simulink model "stepRecovery_compatibility"  (Simulink 8.3)
settings: Solver=ode3  SolverMode=SingleTasking  StartTime=0.0  StopTime="CONFIG.SIMULATION_TIME "  FixedStep=CONFIG.Ts  RelTol=1e-3
InitFcn:
  | cd(fileparts(which(bdroot)));
  | initStepRecovery;
values from neighbouring files (symbols this model uses):
  baseToWorldRotationPort = '/matlabTorqueBalancing/floatingBaseRotationMatrix:i'    [esperimento_fake2.mat]    (also in initStepRecovery.m = ['/' WBT_modelName '/floatingBaseRotationMatrix:i']; initTorqueBalancing.m = ['/' WBT_modelName '/floatingBaseRotationMatrix:i']; secondo_risultato.mat)
  bVectorConstraints = [0 0 0 0 0 0 0 0 0 0 0 0 ... (19 elements, 19x1)]    [esperimento_fake2.mat]    (also in secondo_risultato.mat)
  CONFIG =     [esperimento_fake2.mat]    (also in secondo_risultato.mat)
  ConstraintsMatrix = [3.73205080757 1 0.267949192431 -0.267949192431 -1 -3.73205080757 -3.73205080757 -1 -0.267949192431 0.267949192431 1 3.73205080757 ... (114 elements, 19x6)]    [esperimento_fake2.mat]    (also in secondo_risultato.mat)
  gain =     [esperimento_fake2.mat]    (also in secondo_risultato.mat)
  references =     [esperimento_fake2.mat]    (also in secondo_risultato.mat)
  reg =     [esperimento_fake2.mat]    (also in secondo_risultato.mat)
  ROBOT_DOF = 23    [esperimento_fake2.mat]    (also in secondo_risultato.mat)
  ROBOT_DOF_FOR_SIMULINK = [1 0 0 0 0 0 0 0 0 0 0 0 ... (529 elements, 23x23)]    [esperimento_fake2.mat]    (also in secondo_risultato.mat)
  sat =     [esperimento_fake2.mat]    (also in secondo_risultato.mat)
  SM =     [esperimento_fake2.mat]    (also in secondo_risultato.mat)
  sm =     [esperimento_fake2.mat]    (also in secondo_risultato.mat)
  WBT_modelName = 'matlabTorqueBalancing'    [esperimento_fake2.mat]    (also in initStepRecovery.m; initTorqueBalancing.m; secondo_risultato.mat)
  WBT_robotName = ''    [esperimento_fake2.mat]    (also in secondo_risultato.mat)
undefined symbols (not defined in the file or in its folder): bVectorConstraintsMPC, ConstraintsMatrixMPC, DiscIntNeverNeededParam, mpc_init
libraries: WBToolboxLibrary x191, simulink x22, simulink_extras x4
(part 5 of 6)

== system stepRecovery_compatibility/DesValues/State Machine Step Recovery/Step Recovery reference generator/Step Recovery Techniques /FPE module ==
  foot_x : Inport
  COM_velocity : Inport  Port=2
  COMx : Inport  Port=3
  Joint Configuration : Inport  Port=4
  Base Pose : Inport  Port=5
  Constraints : Inport  Port=6
  Base Pose1 : InportShadow  Port=5
  "CoM6D ->  CoMXYZ2" : Selector  NumberOfDimensions=2  InputPortWidth=7  IndexOptions=Index vector (dialog),Index vector (dialog)  Indices=[1 2 3],[4]  OutputSizes=1,1
  Constant1 : Constant  Value=9.81
  Constant3 : Constant  Value=CONFIG.SR.FPE.offset
  J_COM : Selector  NumberOfDimensions=2  InputPortWidth=3  IndexOptions=Index vector (dialog),Index vector (dialog)  Indices=[4:6],[4:6]  OutputSizes=1,1
  Joint Configuration1 : InportShadow  Port=4
  MATLAB Function : MATLAB Function  TreatAsAtomicUnit=on
      settings: PermitHierarchicalResolution=ParametersOnly
  MATLAB Function2 : MATLAB Function  TreatAsAtomicUnit=on
      settings: PermitHierarchicalResolution=ParametersOnly
  Mass Matrix : WBToolboxLibrary/wholeBodyModel/Dynamics/Mass Matrix  robotName=WBT_robotName  localName=WBT_modelName  wbiFile=WBT_wbiFilename  wbiList=WBT_wbiList
  Mbb : Selector  NumberOfDimensions=2  InputPortWidth=3  IndexOptions=Index vector (dialog),Index vector (dialog)  Indices=[1:6],[1:6]  OutputSizes=1,1
  Out of left foot_CH : Subsystem
  Scope2 : Scope
      settings: TimeRange=auto  MaxDataPoints=5000  SaveToWorkspace=off  YMin=0.9762  YMax=1.00264  SampleTime=-1
  Switch : Switch  Criteria=u2 > Threshold
  To Workspace : ToWorkspace  VariableName=dissipation  SampleTime=-1
  mass : Selector  NumberOfDimensions=2  InputPortWidth=3  IndexOptions=Index vector (dialog),Index vector (dialog)  Indices=[1],[1]  OutputSizes=1,1
  FPE : Outport
  OUT_L : Outport  Port=2
  Direction : Outport  Port=3
  FPE_ORIGINAL : Outport  Port=4
  theta_bar : Outport  Port=5
  OUT_REAL : Outport  Port=6
  OUT_CH : Outport  Port=7
  wires:
  Mass Matrix/1 -> Mbb/1
  Base Pose/1 -> "CoM6D ->  CoMXYZ2"/1, Mass Matrix/1
  Joint Configuration/1 -> Mass Matrix/2
  Mbb/1 -> MATLAB Function/2(Mbb)
  MATLAB Function/1(Mbb_COM) -> J_COM/1, mass/1
  "CoM6D ->  CoMXYZ2"/1 -> MATLAB Function/1(base_origin)
  COM_velocity/1 -> MATLAB Function2/1(COM_vel)
  mass/1 -> MATLAB Function2/2(m)
  COMx/1 -> MATLAB Function/3(COMx), MATLAB Function2/4(COMx)
  Constant1/1 -> MATLAB Function2/5(g)
  MATLAB Function2/1(theta_bar) -> theta_bar/1
  foot_x/1 -> MATLAB Function2/6(foot)
  MATLAB Function2/2(x) -> Direction/1
  MATLAB Function2/3(fpe_poly) -> Out of left foot_CH/1(X_global), Switch/3, FPE_ORIGINAL/1
  Base Pose1/1 -> Out of left foot_CH/3(w_H_base)
  Joint Configuration1/1 -> Out of left foot_CH/2(qj)
  Constraints/1 -> Out of left foot_CH/4(Constraints)
  Out of left foot_CH/1(OUT_L) -> Switch/2, OUT_L/1
  Out of left foot_CH/2(OUT_CH) -> OUT_CH/1
  Out of left foot_CH/3(OUT_REAL) -> OUT_REAL/1
  MATLAB Function2/4(fpe_poly_offset) -> Switch/1
  Switch/1 -> FPE/1
  MATLAB Function2/5(dissipation) -> To Workspace/1, Scope2/1
  Constant3/1 -> MATLAB Function2/7(offset)
  J_COM/1 -> MATLAB Function2/3(J_COM)

== system stepRecovery_compatibility/DesValues/State Machine Step Recovery/Step Recovery reference generator/Step Recovery Techniques /ankle, CoP, Cmp (LEFT FOOT) ==
  Contact_Wrench : Inport
  CoMx : Inport  Port=2
  w_H_lsole : Inport  Port=3
  CMP computer : Subsystem
  COP computer : Subsystem
  Constant : Constant
  Matrix Multiply : Product  Multiplication=Matrix(*)
  Mux1 : Mux  Inputs=2
  Selector : Selector  NumberOfDimensions=2  InputPortWidth=3  IndexOptions=Index vector (dialog),Index vector (dialog)  Indices=[1: 3],4  OutputSizes=1,1
  Selector1 : Selector  InputPortWidth=4  IndexOptions=Index vector (dialog)  Indices=[1:3]  OutputSizes=1
  Sum1 : Sum  Inputs=-+|
  xAnkle : Outport
  CoP : Outport  Port=2
  deltaCoP : Outport  Port=3
  r_CMP : Outport  Port=4
  deltaCMP : Outport  Port=5
  wires:
  Constant/1 -> Mux1/2
  w_H_lsole/1 -> CMP computer/1(w_H_l), Matrix Multiply/1, Selector/1
  Mux1/1 -> Matrix Multiply/2
  Matrix Multiply/1 -> Selector1/1
  COP computer/1(DeltaR_Cop) -> deltaCoP/1, Mux1/1
  Selector/1 -> Sum1/1, xAnkle/1
  Selector1/1 -> CoP/1
  Contact_Wrench/1 -> CMP computer/2(Contact Wrench), COP computer/1(Contact Wrench)
  CMP computer/1(R_CMP) -> r_CMP/1, Sum1/2
  Sum1/1 -> deltaCMP/1
  CoMx/1 -> CMP computer/3(COM position)

== system stepRecovery_compatibility/DesValues/State Machine Step Recovery/visualise inertial/l_sole_H_root_link2/Visualize hom transf4 ==
  H : Inport
  "CoM6D ->  CoMXYZ1" : Selector  NumberOfDimensions=2  InputPortWidth=7  IndexOptions=Index vector (dialog),Index vector (dialog)  Indices=[1 2 3],[1 2 3]  OutputSizes=1,1
  "CoM6D ->  CoMXYZ2" : Selector  NumberOfDimensions=2  InputPortWidth=7  IndexOptions=Index vector (dialog),Index vector (dialog)  Indices=[1 2 3],[4]  OutputSizes=1,1
  Hom : Scope
      settings: TimeRange=auto  ShowLegends=on  MaxDataPoints=5000  SaveToWorkspace=off  SaveName=ScopeData3  YMin=-1.25  YMax=1.25  SampleTime=-1
  R : Scope
      settings: TimeRange=auto  MaxDataPoints=5000  SaveToWorkspace=off  YMin=-0.125  YMax=1.125  SampleTime=-1
  p : Scope
      settings: TimeRange=auto  MaxDataPoints=5000  SaveToWorkspace=off  SaveName=ScopeData2  YMin=-1.00000  YMax=1.00000  SampleTime=-1
  wires:
  H/1 -> "CoM6D ->  CoMXYZ1"/1, Hom/1, "CoM6D ->  CoMXYZ2"/1
  "CoM6D ->  CoMXYZ2"/1 -> p/1
  "CoM6D ->  CoMXYZ1"/1 -> R/1

== system stepRecovery_compatibility/DesValues/State Machine Step Recovery/visualise inertial/l_sole_H_root_link3/Visualize hom transf4 ==
  H : Inport
  "CoM6D ->  CoMXYZ1" : Selector  NumberOfDimensions=2  InputPortWidth=7  IndexOptions=Index vector (dialog),Index vector (dialog)  Indices=[1 2 3],[1 2 3]  OutputSizes=1,1
  "CoM6D ->  CoMXYZ2" : Selector  NumberOfDimensions=2  InputPortWidth=7  IndexOptions=Index vector (dialog),Index vector (dialog)  Indices=[1 2 3],[4]  OutputSizes=1,1
  Hom : Scope
      settings: TimeRange=auto  ShowLegends=on  MaxDataPoints=5000  SaveToWorkspace=off  SaveName=ScopeData3  YMin=-1.25  YMax=1.25  SampleTime=-1
  R : Scope
      settings: TimeRange=auto  MaxDataPoints=5000  SaveToWorkspace=off  YMin=-0.125  YMax=1.125  SampleTime=-1
  p : Scope
      settings: TimeRange=auto  MaxDataPoints=5000  SaveToWorkspace=off  SaveName=ScopeData2  YMin=-1.00000  YMax=1.00000  SampleTime=-1
  wires:
  H/1 -> "CoM6D ->  CoMXYZ1"/1, Hom/1, "CoM6D ->  CoMXYZ2"/1
  "CoM6D ->  CoMXYZ2"/1 -> p/1
  "CoM6D ->  CoMXYZ1"/1 -> R/1

== system stepRecovery_compatibility/DesValues/State Machine Step Recovery/Step Recovery reference generator/Inverse Kinematics/Pseudo-Inverse kinematics Solver/From guess to q_ikin ==
  constraints : Inport
  w_H_b : Inport  Port=2
  q0 : Inport  Port=3
  "qGuess " : Inport  Port=4
  Changed1 : Subsystem
  Constant : Constant  Value=eye(4)
  Constant1 : Constant  Value=eye(4)
  Demux : Demux  Outputs=2
  Demux1 : Demux  Outputs=2
  Forward Kinematics : WBToolboxLibrary/wholeBodyModel/Kinematics/Forward Kinematics  frameName='l_sole'  robotName=WBT_robotName  localName=WBT_modelName  wbiFile=WBT_wbiFilename  wbiList=WBT_wbiList
  Forward Kinematics1 : WBToolboxLibrary/wholeBodyModel/Kinematics/Forward Kinematics  frameName='r_sole'  robotName=WBT_robotName  localName=WBT_modelName  wbiFile=WBT_wbiFilename  wbiList=WBT_wbiList
  MATLAB Function1 : MATLAB Function  TreatAsAtomicUnit=on
      settings: PermitHierarchicalResolution=ParametersOnly
  Matrix Multiply : Product  Multiplication=Matrix(*)
  Mux1 : Mux  Inputs=2
  Reshape1 : Reshape
  Switch{,1..3} (4 alike) : Switch  Criteria=u2 > Threshold
  l_sole_H_root_link1 : Subsystem  mask{link_name='r_sole'}
  l_sole_H_root_link2 : Subsystem  mask{link_name='l_sole'}
  q_ikin_guess : Outport
  wires:
  w_H_b/1 -> Forward Kinematics1/1, Forward Kinematics/1
  q0/1 -> Forward Kinematics/2, Forward Kinematics1/2
  Forward Kinematics/1 -> Switch/1
  Demux/1 -> Switch/2
  Forward Kinematics1/1 -> Switch1/1
  Demux/2 -> Switch1/2
  Switch1/1 -> Switch/3
  Switch/1 -> MATLAB Function1/1(s)
  Constant/1 -> Switch1/3
  Mux1/1 -> q_ikin_guess/1
  Changed1/1(OUT) -> MATLAB Function1/2(reset)
  "qGuess "/1 -> l_sole_H_root_link1/1(qj), Mux1/2, l_sole_H_root_link2/1(qj)
  constraints/1 -> Demux1/1, Changed1/1(IN), Demux/1
  l_sole_H_root_link2/1(link_name_H_root_link) -> Switch2/1
  Demux1/1 -> Switch2/2
  l_sole_H_root_link1/1(link_name_H_root_link) -> Switch3/1
  Demux1/2 -> Switch3/2
  Switch3/1 -> Switch2/3
  Switch2/1 -> Matrix Multiply/2  "contsraint_H_base"
  Constant1/1 -> Switch3/3
  Reshape1/1 -> Mux1/1
  MATLAB Function1/1(s0) -> Matrix Multiply/1  "w_H_constraints"
  Matrix Multiply/1 -> Reshape1/1  "w_H_b"

== system stepRecovery_compatibility/DesValues/State Machine Step Recovery/Step Recovery reference generator/Inverse Kinematics/Pseudo-Inverse kinematics Solver/Generate ikin Errors ==
  CoMrefsDes : Inport
  posturesDes : Inport  Port=2
  Jlfoot : Inport  Port=3
  Jrfoot : Inport  Port=4
  JCoM : Inport  Port=5
  rfootPos : Inport  Port=6
  lfootPos : Inport  Port=7
  CoMPos : Inport  Port=8
  lfootOri : Inport  Port=9
  rfootOri : Inport  Port=10
  NuRef_iKin : Inport  Port=11
  qRef_ikin : Inport  Port=12
  cartesian_err : Inport  Port=13
  "CoM6D ->  CoMXYZ1" : Selector  InputPortWidth=6  IndexOptions=Index vector (dialog)  Indices=[1 2 3]  OutputSizes=1
  Demux1 : Demux  Outputs=[6,ROBOT_DOF]
  Demux2 : Demux  Outputs=[16,ROBOT_DOF]
  JcNu : Product  Multiplication=Matrix(*)
  JcNu1 : Product  Multiplication=Matrix(*)
  JcNu2 : Product  Multiplication=Matrix(*)
  Terminator : Terminator
  Terminator1 : Terminator
  trajectoryGeneratorCoM : MATLAB Function  TreatAsAtomicUnit=on
      settings: PermitHierarchicalResolution=ParametersOnly
  iKinFeetCorr : Outport
  iKinComCorr : Outport  Port=2
  iKinSoleCorr : Outport  Port=3
  iKinPostCorr : Outport  Port=4
  wires:
  Jrfoot/1 -> JcNu1/1
  trajectoryGeneratorCoM/1(iKinFeetCorr) -> iKinFeetCorr/1
  Demux1/1 -> Terminator/1
  CoMPos/1 -> trajectoryGeneratorCoM/6(xCoM)
  trajectoryGeneratorCoM/2(iKinComCorr) -> iKinComCorr/1
  Jlfoot/1 -> JcNu2/1
  CoMrefsDes/1 -> trajectoryGeneratorCoM/8(CoMRefsDes)
  JcNu/1 -> "CoM6D ->  CoMXYZ1"/1
  lfootPos/1 -> trajectoryGeneratorCoM/1(lFootPos)
  trajectoryGeneratorCoM/4(iKinPostCorr) -> iKinPostCorr/1
  JCoM/1 -> JcNu/1
  rfootPos/1 -> trajectoryGeneratorCoM/2(rFootPos)
  NuRef_iKin/1 -> JcNu1/2, Demux1/1, JcNu/2, JcNu2/2
  rfootOri/1 -> trajectoryGeneratorCoM/3(rFootOri)
  lfootOri/1 -> trajectoryGeneratorCoM/4(lFootOri)
  posturesDes/1 -> trajectoryGeneratorCoM/9(posturesDes)
  JcNu2/1 -> trajectoryGeneratorCoM/10(lFootVel)
  JcNu1/1 -> trajectoryGeneratorCoM/11(rFootVel)
  "CoM6D ->  CoMXYZ1"/1 -> trajectoryGeneratorCoM/12(dxCoM)
  Demux1/2 -> trajectoryGeneratorCoM/13(dqj)
  qRef_ikin/1 -> Demux2/1
  Demux2/1 -> Terminator1/1
  Demux2/2 -> trajectoryGeneratorCoM/7(qj)
  trajectoryGeneratorCoM/3(iKinSoleCorr) -> iKinSoleCorr/1
  cartesian_err/1 -> trajectoryGeneratorCoM/5(cartesian_error)

== system stepRecovery_compatibility/DesValues/State Machine Step Recovery/Step Recovery reference generator/Inverse Kinematics/Pseudo-Inverse kinematics Solver/ikin visualizer ==
  Ikin_feetCorr : Inport
  Ikin_CoMCorr : Inport  Port=2
  Ikin_PostCorr : Inport  Port=3
  ikin_sole_Corr : Inport  Port=4
  CoM Desired Dynamics : Scope
      settings: TimeRange=auto  MaxDataPoints=5000  SaveToWorkspace=off  SaveName=ScopeData  YMin=-3.74023  YMax=13.04104  SampleTime=-1
  Demux : Demux  Outputs=2
  Demux1 : Demux  Outputs=[3,4,4,6,6]
  Feet Desired Dynamics : Scope
      settings: TimeRange=auto  MaxDataPoints=5000  SaveToWorkspace=off  YMin=-11.5408  YMax=11.5143  SampleTime=-1
  Scope : Scope  NumInputPorts=5
      settings: TimeRange=auto  MaxDataPoints=5000  SaveToWorkspace=off  YMin=-10~-10~-10~-10~-10  YMax=10~10~10~10~10  SampleTime=-1
  desired foot positioning : Scope  NumInputPorts=2
      settings: TimeRange=auto  ShowLegends=on  MaxDataPoints=5000  SaveToWorkspace=off  SaveName=ScopeData2  YMin=-139.12636~-22.83526  YMax=38.44709~32.38622  SampleTime=-1
  wires:
  Ikin_CoMCorr/1 -> CoM Desired Dynamics/1
  Ikin_feetCorr/1 -> Feet Desired Dynamics/1
  Ikin_PostCorr/1 -> Demux1/1
  ikin_sole_Corr/1 -> Demux/1
  Demux/1 -> desired foot positioning/1  "left foot (cartesian)"
  Demux/2 -> desired foot positioning/2  "right foot (cartesian)"
  Demux1/1 -> Scope/1  "torso"
  Demux1/2 -> Scope/2  "left arm"
  Demux1/3 -> Scope/3  "right arm"
  Demux1/4 -> Scope/4  "left leg"
  Demux1/5 -> Scope/5  "right leg"

== system stepRecovery_compatibility/DesValues/State Machine Step Recovery/Step Recovery reference generator/Inverse Kinematics/Pseudo-Inverse kinematics Solver/ikin_DoubleIntegrator ==
  dNuRef_ikin : Inport
  Nu_ikin_init : Inport  Port=2
  q_guess : Inport  Port=3
  Acceleration Integration : DiscreteIntegrator  ExternalReset=rising  InitialConditionSource=external  SampleTime=CONFIG.Ts  ICPrevOutput=DiscIntNeverNeededParam  ICPrevScaledInput=DiscIntNeverNeededParam
  BaseDerivative : MATLAB Function  TreatAsAtomicUnit=on
      settings: PermitHierarchicalResolution=ParametersOnly
  Changed : Subsystem
  Changed1 : Subsystem
  Define the base pose as pos+quat : MATLAB Function  TreatAsAtomicUnit=on
      settings: PermitHierarchicalResolution=ParametersOnly
  Define the base pose as transformation matrix : MATLAB Function  TreatAsAtomicUnit=on
      settings: PermitHierarchicalResolution=ParametersOnly
  Demux : Demux  Outputs=[7;ROBOT_DOF]
  Demux1 : Demux  Outputs=[6;ROBOT_DOF]
  Demux2 : Demux  Outputs=[16,ROBOT_DOF]
  Joints references : MATLAB Function  TreatAsAtomicUnit=on
      settings: PermitHierarchicalResolution=ParametersOnly
  Mux : Mux  Inputs=2
  Terminator : Terminator
  Terminator1 : Terminator
  Velocity Integration : DiscreteIntegrator  ExternalReset=rising  InitialConditionSource=external  SampleTime=CONFIG.Ts  ICPrevOutput=DiscIntNeverNeededParam  ICPrevScaledInput=DiscIntNeverNeededParam
  NuRef_ikin : Outport
  qRef_ikin : Outport  Port=2
  inverseKinRef : Outport  Port=3
  qjRef_ikin : Outport  Port=4
  wires:
  Nu_ikin_init/1 -> Acceleration Integration/3, Changed/1(IN)
  q_guess/1 -> Define the base pose as pos+quat/1(qRef_ikin_init)
  dNuRef_ikin/1 -> Joints references/1(dNuRef_ikin), Acceleration Integration/1
  Demux/2 -> Terminator/1
  Demux/1 -> BaseDerivative/2(baseQuat)
  Velocity Integration/1 -> Define the base pose as transformation matrix/1(qRef_ikin_no_converted), Demux/1, Joints references/3(qRef_ikin)
  Acceleration Integration/1 -> Joints references/2(NuRef_ikin), Demux1/1, NuRef_ikin/1
  Demux1/1 -> BaseDerivative/1(NuBase_Ref)
  BaseDerivative/1(BaseDer) -> Mux/1
  Demux1/2 -> Mux/2
  Mux/1 -> Velocity Integration/1
  Joints references/1(inverseKinRef) -> inverseKinRef/1
  Define the base pose as transformation matrix/1(qRef_ikin) -> Demux2/1, qRef_ikin/1
  Define the base pose as pos+quat/1(qRef_ikin_0) -> Changed1/1(IN), Velocity Integration/3
  Demux2/2 -> qjRef_ikin/1
  Demux2/1 -> Terminator1/1
  Changed1/1(OUT) -> Velocity Integration/2
  Changed/1(OUT) -> Acceleration Integration/2

== system stepRecovery_compatibility/DesValues/State Machine Step Recovery/Step Recovery reference generator/Inverse Kinematics/Pseudo-Inverse kinematics Solver/ikin_utilities ==
  lsole_H_rsole : Inport
  rsole_H_lsole : Inport  Port=2
  qRef_ikin : Inport  Port=3
  NuRef_ikin : Inport  Port=4
  qRef_ikin_init : Inport  Port=5
  ikin_Jacobians : Subsystem
  ikin_dJNu : Subsystem
  ikin_forwardKin : Subsystem
  Jlsole : Outport
  Jrsole : Outport  Port=2
  JCoM : Outport  Port=3
  deltaRFootPos : Outport  Port=4
  deltaLFootPos : Outport  Port=5
  CoMPos : Outport  Port=6
  deltaLFootOri : Outport  Port=7
  deltaRFootOri : Outport  Port=8
  cartesian_err : Outport  Port=9
  dJlfootNu : Outport  Port=10
  dJrfootNu : Outport  Port=11
  dJCoMNu : Outport  Port=12
  wires:
  ikin_Jacobians/1(Jlsole) -> Jlsole/1
  ikin_Jacobians/3(JCoM) -> JCoM/1
  ikin_dJNu/3(dJCoMNu) -> dJCoMNu/1
  ikin_dJNu/1(dJlfootNu) -> dJlfootNu/1
  ikin_dJNu/2(dJrfootNu) -> dJrfootNu/1
  ikin_Jacobians/2(Jrsole) -> Jrsole/1
  qRef_ikin_init/1 -> ikin_forwardKin/1(qRef_iKin_init)
  qRef_ikin/1 -> ikin_Jacobians/1(qRef_iKin), ikin_forwardKin/2(qRef_iKin), ikin_dJNu/2(qRef_iKin)
  ikin_forwardKin/1(CoMpos) -> CoMPos/1
  ikin_forwardKin/2(deltaLFootPos) -> deltaLFootPos/1
  ikin_forwardKin/3(deltaRFootOri) -> deltaRFootOri/1
  ikin_forwardKin/4(deltaRFootPos) -> deltaRFootPos/1
  ikin_forwardKin/5(deltaLFootOri) -> deltaLFootOri/1
  NuRef_ikin/1 -> ikin_dJNu/1(NuRef_iKin)
  lsole_H_rsole/1 -> ikin_forwardKin/3(lsole_H_rsole)
  rsole_H_lsole/1 -> ikin_forwardKin/4("rsole_H_lsole ")
  ikin_forwardKin/6(cartesian_err) -> cartesian_err/1

== system stepRecovery_compatibility/DesValues/State Machine Step Recovery/Step Recovery reference generator/Inverse Kinematics/Pseudo-Inverse kinematics Solver/q+base ==
  note: This is used to keep the foot still since the last time constraints changed.
      | Indeed it is not updated at every time instant otherwise is the foot starts rotating in the menwhile, the IK does not keep that rotation.
      | Therefore here it is assumed that the stnace foot (feet) is (are) well placed when the constraints vector changes.
  qj : Inport
  w_H_b : Inport  Port=2
  constraints : Inport  Port=3
  Changed1 : Subsystem
  MATLAB Function1 : MATLAB Function  TreatAsAtomicUnit=on
      settings: PermitHierarchicalResolution=ParametersOnly
  Mux4 : Mux  Inputs=2
  Reshape1 : Reshape
  qRef_ikin_ini : Outport
  wires:
  Reshape1/1 -> Mux4/1
  w_H_b/1 -> Reshape1/1
  qj/1 -> Mux4/2
  Mux4/1 -> MATLAB Function1/1(s)
  MATLAB Function1/1(s0) -> qRef_ikin_ini/1
  Changed1/1(OUT) -> MATLAB Function1/2(reset)
  constraints/1 -> Changed1/1(IN)

== system stepRecovery_compatibility/DesValues/State Machine Step Recovery/Step Recovery reference generator/Step Recovery Techniques /Capture Point Computer/Capture Point ==
  STATE : Inport
  r_CxP : Inport  Port=2
  COMx : Inport  Port=3
  r_icp : Inport  Port=4
  OUT : Inport  Port=5
  OUT_CH : Inport  Port=6
  Compare To Constant : simulink/Logic and Bit Operations/Compare To Constant  relop===  const=14  OutDataTypeStr=boolean
  Constant : Constant  Value=CONFIG.Ts
  Constant1 : Constant  Value=CONFIG.SR.CP.robotStepTime
  Constant4 : Constant  Value=gain.ik_offset+[0.02;0;0]
  Data Type Conversion : DataTypeConversion  OutDataTypeStr=boolean
  Data Type Conversion2 : DataTypeConversion  OutDataTypeStr=double
  Logical Operator : Logic  Operator=NOR  AllPortsSameDT=off  OutDataTypeStr=boolean
  MATLAB Function : MATLAB Function  TreatAsAtomicUnit=on
      settings: PermitHierarchicalResolution=ParametersOnly
  MATLAB Function1 : MATLAB Function  TreatAsAtomicUnit=on
      settings: PermitHierarchicalResolution=ParametersOnly
  Mux : Mux
  Product : Product
  S-R Flip-Flop : simulink_extras/Flip Flops/S-R Flip-Flop  initial_condition=0
  Sum : Sum  Inputs=++|
  Versor : MATLAB Function  TreatAsAtomicUnit=on
      settings: PermitHierarchicalResolution=ParametersOnly
  omega : Subsystem
  r_icp1 : InportShadow  Port=4
  "r_CP " : Outport
  "STEP " : Outport  Port=2
  Direction : Outport  Port=3
  CoP_ref : Outport  Port=4
  wires:
  Data Type Conversion/1 -> S-R Flip-Flop/1
  r_CxP/1 -> Versor/1(r_CxP), MATLAB Function1/2(r)
  S-R Flip-Flop/1 -> Data Type Conversion2/1
  omega/1(omega) -> Versor/2(omega), MATLAB Function/1(omega), MATLAB Function1/1(omega)
  Constant/1 -> MATLAB Function1/3(delta_t)
  COMx/1 -> omega/1(COMx)
  MATLAB Function1/1(r_eq) -> MATLAB Function/3(r_CxP)
  Constant1/1 -> MATLAB Function/4(robot_step_time)
  MATLAB Function/1(r_CP) -> Sum/2, "r_CP "/1
  Data Type Conversion2/1 -> "STEP "/1, MATLAB Function/5(STEP), Mux/4, Product/2, MATLAB Function1/4(OUT)
  r_icp/1 -> Versor/3(r_ic), MATLAB Function/2(r_ic)
  Versor/1(r_ic_dot) -> Direction/1
  Logical Operator/1 -> S-R Flip-Flop/2
  OUT/1 -> Data Type Conversion/1
  STATE/1 -> Compare To Constant/1
  Compare To Constant/1 -> Logical Operator/2
  OUT_CH/1 -> Logical Operator/1
  MATLAB Function/2(r_ic0) -> Mux/2
  r_icp1/1 -> Mux/3
  Mux/1 -> CoP_ref/1
  Sum/1 -> Mux/1
  Constant4/1 -> Product/1
  Product/1 -> Sum/1

== system stepRecovery_compatibility/DesValues/State Machine Step Recovery/Step Recovery reference generator/Step Recovery Techniques /Capture Point Computer/Capture Point-Pratt  ==
  w_H_f : Inport
  STATE : Inport  Port=2
  COMx : Inport  Port=3
  r_icp : Inport  Port=4
  OUT : Inport  Port=5
  OUT_CH : Inport  Port=6
  Compare To Constant : simulink/Logic and Bit Operations/Compare To Constant  relop===  const=14  OutDataTypeStr=boolean
  Constant1 : Constant  Value=CONFIG.SR.CP.robotStepTime
  Constant3 : Constant  Value=gain.footSize_step
  Data Type Conversion : DataTypeConversion  OutDataTypeStr=boolean
  Data Type Conversion2 : DataTypeConversion  OutDataTypeStr=double
  Logical Operator : Logic  Operator=NOR  AllPortsSameDT=off  OutDataTypeStr=boolean
  MATLAB Function : MATLAB Function  TreatAsAtomicUnit=on
      settings: PermitHierarchicalResolution=ParametersOnly
  S-R Flip-Flop : simulink_extras/Flip Flops/S-R Flip-Flop  initial_condition=0
  Scope : Scope
      settings: TimeRange=auto  MaxDataPoints=5000  SaveToWorkspace=off  YMin=-1.00000  YMax=1.00000  SampleTime=-1
  Scope1 : Scope
      settings: TimeRange=auto  MaxDataPoints=5000  SaveToWorkspace=off  SaveName=ScopeData2  YMin=-1.00000  YMax=1.00000  SampleTime=-1
  omega : Subsystem
  "r_CP " : Outport
  "STEP " : Outport  Port=2
  wires:
  Compare To Constant/1 -> Logical Operator/2
  STATE/1 -> Compare To Constant/1
  OUT_CH/1 -> Logical Operator/1
  Logical Operator/1 -> S-R Flip-Flop/2
  OUT/1 -> Data Type Conversion/1
  Data Type Conversion/1 -> S-R Flip-Flop/1
  S-R Flip-Flop/1 -> Data Type Conversion2/1
  omega/1(omega) -> MATLAB Function/1(omega)
  COMx/1 -> omega/1(COMx)
  r_icp/1 -> MATLAB Function/2(r_ic)
  Constant1/1 -> MATLAB Function/3(robot_step_time)
  MATLAB Function/1(r_CP) -> "r_CP "/1
  Data Type Conversion2/1 -> "STEP "/1, MATLAB Function/4(STEP)
  w_H_f/1 -> MATLAB Function/5(w_H_f)
  Constant3/1 -> MATLAB Function/6(foot_size)
  MATLAB Function/2(T1) -> Scope/1
  MATLAB Function/3(T2) -> Scope1/1

== system stepRecovery_compatibility/DesValues/State Machine Step Recovery/Step Recovery reference generator/Step Recovery Techniques /Capture Point Computer/Capture Point-alternative ==
  STATE : Inport
  r_CxP : Inport  Port=2
  COMx : Inport  Port=3
  r_icp : Inport  Port=4
  OUT : Inport  Port=5
  OUT_CH : Inport  Port=6
  Compare To Constant : simulink/Logic and Bit Operations/Compare To Constant  relop===  const=14  OutDataTypeStr=boolean
  Constant1 : Constant  Value=CONFIG.SR.CP.robotStepTime
  Constant2 : Constant  Value=CONFIG.Ts
  Data Type Conversion : DataTypeConversion  OutDataTypeStr=boolean
  Data Type Conversion2 : DataTypeConversion  OutDataTypeStr=double
  Logical Operator : Logic  Operator=NOR  AllPortsSameDT=off  OutDataTypeStr=boolean
  MATLAB Function : MATLAB Function  TreatAsAtomicUnit=on
      settings: PermitHierarchicalResolution=ParametersOnly
  S-R Flip-Flop : simulink_extras/Flip Flops/S-R Flip-Flop  initial_condition=0
  omega : Subsystem
  "r_CP " : Outport
  "STEP " : Outport  Port=2
  wires:
  Constant2/1 -> MATLAB Function/6(delta_t)
  Data Type Conversion2/1 -> MATLAB Function/5(STEP), "STEP "/1
  MATLAB Function/1(r_CP) -> "r_CP "/1
  Constant1/1 -> MATLAB Function/4(robot_step_time)
  r_icp/1 -> MATLAB Function/2(r_ic)
  r_CxP/1 -> MATLAB Function/3(r_CxP)
  COMx/1 -> omega/1(COMx)
  omega/1(omega) -> MATLAB Function/1(omega)
  S-R Flip-Flop/1 -> Data Type Conversion2/1
  Data Type Conversion/1 -> S-R Flip-Flop/1
  OUT/1 -> Data Type Conversion/1
  Logical Operator/1 -> S-R Flip-Flop/2
  OUT_CH/1 -> Logical Operator/1
  STATE/1 -> Compare To Constant/1
  Compare To Constant/1 -> Logical Operator/2

== system stepRecovery_compatibility/DesValues/State Machine Step Recovery/Step Recovery reference generator/Step Recovery Techniques /Capture Point Computer/ICP  ==
  note: Instantaneous capture point
  COM position : Inport
  COM velocity : Inport  Port=2
  Divide1 : Product  Inputs=/*
  Sum : Sum  Inputs=|++
  omega : Subsystem
  zero height : Gain  Gain=[1,0,0;0,1,0;0,0,0]  Multiplication=Matrix(K*u)
  icp : Outport
  wires:
  COM position/1 -> omega/1(COMx), Sum/1
  Divide1/1 -> Sum/2
  COM velocity/1 -> Divide1/2
  Sum/1 -> zero height/1
  zero height/1 -> icp/1
  omega/1(omega) -> Divide1/1

== system stepRecovery_compatibility/DesValues/State Machine Step Recovery/Step Recovery reference generator/Step Recovery Techniques /Capture Point Computer/Out of left foot_CH ==
  X_global : Inport
  Constraints : Inport  Port=2
  w_H_lsole : Inport  Port=3
  w_H_rsole : Inport  Port=4
  Constant : Constant
  Constant1 : Constant  Value=gain.l_foot_shadowed
  Constant2 : Constant  Value=gain.footSize_step
  Constant3 : Constant  Value=gain.footSize
  Inverse : MATLAB Function  TreatAsAtomicUnit=on
      settings: PermitHierarchicalResolution=ParametersOnly
  MATLAB Function : MATLAB Function  TreatAsAtomicUnit=on
      settings: PermitHierarchicalResolution=ParametersOnly
  Matrix Multiply : Product  Multiplication=Matrix(*)
  Mux : Mux  Inputs=2
  "Out of left foot " : MATLAB Function  TreatAsAtomicUnit=on
      settings: PermitHierarchicalResolution=ParametersOnly
  Selector : Selector  InputPortWidth=2  IndexOptions=Index vector (dialog)  Indices=[2]  OutputSizes=1
  Selector2 : Selector  InputPortWidth=4  IndexOptions=Index vector (dialog)  Indices=[1 2]  OutputSizes=1
  Switch : Switch  Criteria=u2 > Threshold
  OUT_L : Outport
  OUT_CH : Outport  Port=2
  OUT_REAL : Outport  Port=3
  wires:
  Mux/1 -> Matrix Multiply/2
  Selector2/1 -> "Out of left foot "/1(x)
  Matrix Multiply/1 -> Selector2/1
  Constant/1 -> Mux/2
  w_H_lsole/1 -> MATLAB Function/2(w_H_lsole), Inverse/1(w_H_a)
  "Out of left foot "/1(OUT) -> Switch/3, OUT_L/1
  X_global/1 -> MATLAB Function/1(x), Mux/1
  Inverse/1(a_H_w) -> Matrix Multiply/1
  Constant2/1 -> "Out of left foot "/2(support)
  Constant1/1 -> "Out of left foot "/3(shadow)
  Constant3/1 -> MATLAB Function/4(foot_size)
  w_H_rsole/1 -> MATLAB Function/3(w_H_rsole)
  MATLAB Function/1(OUT) -> Switch/1
  Constraints/1 -> Selector/1
  Selector/1 -> Switch/2
  Switch/1 -> OUT_CH/1
  "Out of left foot "/2(OUT_real) -> OUT_REAL/1

== system stepRecovery_compatibility/DesValues/State Machine Step Recovery/Step Recovery reference generator/Step Recovery Techniques /Dump and Visualize SRT /Subsystem ==
  w_H_b : Inport
  COP : Inport  Port=2
  CMP : Inport  Port=3
  com_lin_vel : Inport  Port=4
  nu : Inport  Port=5
  CP : Inport  Port=6
  CP1 : Inport  Port=7
  "CPratt " : Inport  Port=8
  r_icp : Inport  Port=9
  TRIGGER CP : Inport  Port=10
  CH_CP : Inport  Port=11
  FPE : Inport  Port=12
  TRIGGER FPE : Inport  Port=13
  CH_FPE : Inport  Port=14
  To Workspace : ToWorkspace  VariableName=nu  SampleTime=-1
  To Workspace1 : ToWorkspace  VariableName=COM_lin_vel  SampleTime=-1
  To Workspace10 : ToWorkspace  VariableName=OUT_CONVEXHULL_CP  SampleTime=-1
  To Workspace11 : ToWorkspace  VariableName=OUT_CONVEXHULL_FPE  SampleTime=-1
  To Workspace12 : ToWorkspace  VariableName=CPratt  SampleTime=-1
  To Workspace13 : ToWorkspace  VariableName=r_icp  SampleTime=-1
  To Workspace2 : ToWorkspace  VariableName=w_H_b  SampleTime=-1
  To Workspace3 : ToWorkspace  VariableName=CMP  SampleTime=-1
  To Workspace4 : ToWorkspace  VariableName=COP  SampleTime=-1
  To Workspace5 : ToWorkspace  VariableName=FPE  SampleTime=-1
  To Workspace6 : ToWorkspace  VariableName=TRIGGER_FPE  SampleTime=-1
  To Workspace7 : ToWorkspace  VariableName=TRIGGER_CP  SampleTime=-1
  To Workspace8 : ToWorkspace  VariableName=CP  SampleTime=-1
  To Workspace9 : ToWorkspace  VariableName=CP1  SampleTime=-1
  wires:
  COP/1 -> To Workspace4/1
  com_lin_vel/1 -> To Workspace1/1
  CMP/1 -> To Workspace3/1
  w_H_b/1 -> To Workspace2/1
  nu/1 -> To Workspace/1
  FPE/1 -> To Workspace5/1
  CP/1 -> To Workspace8/1
  CH_CP/1 -> To Workspace10/1
  CH_FPE/1 -> To Workspace11/1
  CP1/1 -> To Workspace9/1
  TRIGGER CP/1 -> To Workspace7/1
  TRIGGER FPE/1 -> To Workspace6/1
  "CPratt "/1 -> To Workspace12/1
  r_icp/1 -> To Workspace13/1

== system stepRecovery_compatibility/DesValues/State Machine Step Recovery/Step Recovery reference generator/Step Recovery Techniques /Dump and Visualize SRT /Visualize  ==
  CP : Inport
  CP1 : Inport  Port=2
  "CP_pratt " : Inport  Port=3
  r_icp : Inport  Port=4
  TRIGGER CP : Inport  Port=5
  OUT_REAL_CP : Inport  Port=6
  CH_CP : Inport  Port=7
  FPE : Inport  Port=8
  TRIGGER FPE : Inport  Port=9
  FPE ORIGINAL : Inport  Port=10
  theta_bar : Inport  Port=11
  OUT_REAL_FPE : Inport  Port=12
  CH_FPE : Inport  Port=13
  Mux : Mux  Inputs=3
  Mux2 : Mux  Inputs=3
  Scope : Scope
      settings: TimeRange=auto  LimitDataPoints=on  MaxDataPoints=5000  SaveToWorkspace=off  SaveName=ScopeData3  YMin=-0.21436  YMax=0.07995  SampleTime=-1  DataFormat=Array
  Scope1 : Scope  Commented=on  NumInputPorts=4
      settings: TimeRange=auto  MaxDataPoints=5000  SaveToWorkspace=off  YMin=-0.22678~-0.07924~-0.00993~-0.125  YMax=0.25479~0.03212~0.00677~1.125  SampleTime=-1
  Scope2 : Scope  NumInputPorts=4
      settings: TimeRange=auto  MaxDataPoints=5000  SaveToWorkspace=off  SaveName=ScopeData2  YMin=-0.30351~-0.43259~-0.61146~-0.125  YMax=0.18653~0.28543~0.59275~1.125  SampleTime=-1
  Scope3 : Scope  Commented=on  NumInputPorts=2
      settings: TimeRange=auto  LimitDataPoints=on  MaxDataPoints=5000  SaveToWorkspace=off  YMin=-0.125~-0.125  YMax=1.125~1.125  SampleTime=-1  DataFormat=Array
  TRIGGER FPE_1 : InportShadow  Port=9
  wires:
  TRIGGER CP/1 -> Scope3/1, Mux/1
  CP/1 -> Scope2/1
  CP1/1 -> Scope2/2
  TRIGGER FPE/1 -> Mux/3
  CH_CP/1 -> Mux/2
  CH_FPE/1 -> Mux2/3
  OUT_REAL_CP/1 -> Scope3/2
  FPE ORIGINAL/1 -> Scope1/2
  theta_bar/1 -> Scope1/3
  Mux2/1 -> Scope1/4  "Triggers"
  OUT_REAL_FPE/1 -> Mux2/2
  Mux/1 -> Scope2/4  "Triggers"
  FPE/1 -> Scope1/1
  TRIGGER FPE_1/1 -> Mux2/1
  "CP_pratt "/1 -> Scope2/3
  r_icp/1 -> Scope/1

== system stepRecovery_compatibility/DesValues/State Machine Step Recovery/Step Recovery reference generator/Step Recovery Techniques /FPE module/Out of left foot_CH ==
  X_global : Inport
  qj : Inport  Port=2
  w_H_base : Inport  Port=3
  Constraints : Inport  Port=4
  Constant : Constant
  Constant1 : Constant  Value=gain.l_foot_shadowed
  Constant2 : Constant  Value=gain.footSize_step
  Constant3 : Constant  Value=gain.footSize
  Forward Kinematics1 : WBToolboxLibrary/wholeBodyModel/Kinematics/Forward Kinematics  frameName='l_sole'  robotName=WBT_robotName  localName=WBT_modelName  wbiFile=WBT_wbiFilename  wbiList=WBT_wbiList
  Forward Kinematics2 : WBToolboxLibrary/wholeBodyModel/Kinematics/Forward Kinematics  frameName='l_sole'  robotName=WBT_robotName  localName=WBT_modelName  wbiFile=WBT_wbiFilename  wbiList=WBT_wbiList
  Inverse : MATLAB Function  TreatAsAtomicUnit=on
      settings: PermitHierarchicalResolution=ParametersOnly
  MATLAB Function : MATLAB Function  TreatAsAtomicUnit=on
      settings: PermitHierarchicalResolution=ParametersOnly
  Matrix Multiply : Product  Multiplication=Matrix(*)
  Mux : Mux  Inputs=2
  "Out of left foot " : MATLAB Function  TreatAsAtomicUnit=on
      settings: PermitHierarchicalResolution=ParametersOnly
  Selector : Selector  InputPortWidth=2  IndexOptions=Index vector (dialog)  Indices=[2]  OutputSizes=1
  Selector2 : Selector  InputPortWidth=4  IndexOptions=Index vector (dialog)  Indices=[1 2]  OutputSizes=1
  Switch : Switch  Criteria=u2 > Threshold
  OUT_L : Outport
  OUT_CH : Outport  Port=2
  OUT_REAL : Outport  Port=3
  wires:
  Mux/1 -> Matrix Multiply/2
  w_H_base/1 -> Forward Kinematics2/1, Forward Kinematics1/1
  Selector2/1 -> "Out of left foot "/1(x)
  Matrix Multiply/1 -> Selector2/1
  Constant/1 -> Mux/2
  Forward Kinematics1/1 -> MATLAB Function/2(w_H_lsole), Inverse/1(w_H_a)
  qj/1 -> Forward Kinematics2/2, Forward Kinematics1/2
  "Out of left foot "/1(OUT) -> Switch/3, OUT_L/1
  X_global/1 -> MATLAB Function/1(x), Mux/1
  Inverse/1(a_H_w) -> Matrix Multiply/1
  Constant2/1 -> "Out of left foot "/2(support)
  Constant1/1 -> "Out of left foot "/3(shadow)
  Constant3/1 -> MATLAB Function/4(foot_size)
  Forward Kinematics2/1 -> MATLAB Function/3(w_H_rsole)
  MATLAB Function/1(OUT) -> Switch/1
  Constraints/1 -> Selector/1
  Selector/1 -> Switch/2
  Switch/1 -> OUT_CH/1
  "Out of left foot "/2(OUT_real) -> OUT_REAL/1

== system stepRecovery_compatibility/DesValues/State Machine Step Recovery/Step Recovery reference generator/Step Recovery Techniques /ankle, CoP, Cmp (LEFT FOOT)/CMP computer ==
  note: expressed in global coordinates
  w_H_l : Inport
  Contact Wrench : Inport  Port=2
  COM position : Inport  Port=3
  Demux : Demux  Outputs=3
  Divide : Product  Inputs=*/
  Divide1 : Product  Inputs=*/
  MATLAB Function : MATLAB Function  TreatAsAtomicUnit=on
      settings: PermitHierarchicalResolution=ParametersOnly
  Matrix Multiply : Product  Multiplication=Matrix(*)
  Mux : Mux  Inputs=3
  Product : Product
  Product1 : Product
  Selector : Selector  InputPortWidth=6  IndexOptions=Index vector (dialog)  Indices=[1:3]  OutputSizes=1
  Selector1 : Selector  InputPortWidth=3  IndexOptions=Index vector (dialog)  Indices=[3]  OutputSizes=1
  Selector2 : Selector  NumberOfDimensions=2  InputPortWidth=3  IndexOptions=Index vector (dialog),Index vector (dialog)  Indices=[1:3],1:3  OutputSizes=1,1
  Selector3 : Selector  NumberOfDimensions=2  InputPortWidth=3  IndexOptions=Index vector (dialog),Index vector (dialog)  Indices=[1:3],4  OutputSizes=1,1
  Sum : Sum  Inputs=+-|
  Transpose : PermuteDimensions
  R_CMP : Outport
  wires:
  Divide/1 -> Product/2
  Product/1 -> Mux/1
  Divide1/1 -> Product1/2
  Sum/1 -> R_CMP/1
  Selector/1 -> Demux/1
  Demux/1 -> Divide/1
  Demux/3 -> Divide/2, Divide1/2
  Demux/2 -> Divide1/1
  COM position/1 -> Sum/1, Selector1/1
  Product1/1 -> Mux/2
  Mux/1 -> Sum/2
  Selector1/1 -> Mux/3, Product1/1, Product/1
  w_H_l/1 -> Selector2/1, Selector3/1
  MATLAB Function/1(s_A_b) -> Transpose/1
  Selector2/1 -> MATLAB Function/1(R)
  Selector3/1 -> MATLAB Function/2(p)
  Matrix Multiply/1 -> Selector/1
  Transpose/1 -> Matrix Multiply/1
  Contact Wrench/1 -> Matrix Multiply/2

== system stepRecovery_compatibility/DesValues/State Machine Step Recovery/Step Recovery reference generator/Step Recovery Techniques /ankle, CoP, Cmp (LEFT FOOT)/COP computer ==
  Contact Wrench : Inport
  Constant : Constant  Value=0
  Demux : Demux  Outputs=3
  Divide : Product  Inputs=*/
  Divide1 : Product  Inputs=*/
  Gain : Gain  Gain=-1
  Mux : Mux  Inputs=3
  Selector : Selector  InputPortWidth=6  IndexOptions=Index vector (dialog)  Indices=[3:5]  OutputSizes=1
  DeltaR_Cop : Outport
  wires:
  Demux/3 -> Divide/1
  Demux/1 -> Divide1/2, Divide/2
  Demux/2 -> Divide1/1
  Divide/1 -> Gain/1
  Gain/1 -> Mux/1
  Divide1/1 -> Mux/2
  Constant/1 -> Mux/3
  Mux/1 -> DeltaR_Cop/1
  Selector/1 -> Demux/1
  Contact Wrench/1 -> Selector/1

== system stepRecovery_compatibility/DesValues/State Machine Step Recovery/Step Recovery reference generator/Inverse Kinematics/Pseudo-Inverse kinematics Solver/From guess to q_ikin/Changed1 ==
  note: If the vector changes this block outputs 1, 0 otherwise
  IN : Inport
  Data Type Conversion : DataTypeConversion
  Data Type Conversion1 : DataTypeConversion
  Memory : Memory
  Relational Operator : RelationalOperator  Operator=~=  OutDataTypeStr=boolean
  Sum of Elements : Sum  Inputs=+
  OUT : Outport
  wires:
  Sum of Elements/1 -> Data Type Conversion1/1
  IN/1 -> Memory/1, Relational Operator/2
  Memory/1 -> Relational Operator/1
  Relational Operator/1 -> Data Type Conversion/1
  Data Type Conversion/1 -> Sum of Elements/1
  Data Type Conversion1/1 -> OUT/1

== system stepRecovery_compatibility/DesValues/State Machine Step Recovery/Step Recovery reference generator/Inverse Kinematics/Pseudo-Inverse kinematics Solver/From guess to q_ikin/l_sole_H_root_link1 ==
  qj : Inport
  Constant5 : Constant  Value=eye(4)
  Constant6 : Constant  Value=eye(4)
  Inv\* : Product  Inputs=/*  Multiplication=Matrix(*)
  Visualize hom transf4 : Subsystem
  link_name : WBToolboxLibrary/wholeBodyModel/Kinematics/Forward Kinematics  frameName=link_name  robotName=WBT_robotName  localName=WBT_modelName  wbiFile=WBT_wbiFilename  wbiList=WBT_wbiList
  root_link : WBToolboxLibrary/wholeBodyModel/Kinematics/Forward Kinematics  frameName='root_link'  robotName=WBT_robotName  localName=WBT_modelName  wbiFile=WBT_wbiFilename  wbiList=WBT_wbiList
  link_name_H_root_link : Outport
  wires:
  root_link/1 -> Inv\*/2, Visualize hom transf4/1(H)
  qj/1 -> root_link/2, link_name/2
  Constant6/1 -> root_link/1
  link_name/1 -> Inv\*/1
  Inv\*/1 -> link_name_H_root_link/1  "link_name_H_root_link"
  Constant5/1 -> link_name/1

== system stepRecovery_compatibility/DesValues/State Machine Step Recovery/Step Recovery reference generator/Inverse Kinematics/Pseudo-Inverse kinematics Solver/From guess to q_ikin/l_sole_H_root_link2 ==
  qj : Inport
  Constant5 : Constant  Value=eye(4)
  Constant6 : Constant  Value=eye(4)
  Inv\* : Product  Inputs=/*  Multiplication=Matrix(*)
  Visualize hom transf4 : Subsystem
  link_name : WBToolboxLibrary/wholeBodyModel/Kinematics/Forward Kinematics  frameName=link_name  robotName=WBT_robotName  localName=WBT_modelName  wbiFile=WBT_wbiFilename  wbiList=WBT_wbiList
  root_link : WBToolboxLibrary/wholeBodyModel/Kinematics/Forward Kinematics  frameName='root_link'  robotName=WBT_robotName  localName=WBT_modelName  wbiFile=WBT_wbiFilename  wbiList=WBT_wbiList
  link_name_H_root_link : Outport
  wires:
  root_link/1 -> Inv\*/2, Visualize hom transf4/1(H)
  qj/1 -> root_link/2, link_name/2
  Constant6/1 -> root_link/1
  link_name/1 -> Inv\*/1
  Inv\*/1 -> link_name_H_root_link/1  "link_name_H_root_link"
  Constant5/1 -> link_name/1

== system stepRecovery_compatibility/DesValues/State Machine Step Recovery/Step Recovery reference generator/Inverse Kinematics/Pseudo-Inverse kinematics Solver/ikin_DoubleIntegrator/Changed ==
  note: If the vector changes this block outputs 1, 0 otherwise
  IN : Inport
  Data Type Conversion : DataTypeConversion
  Data Type Conversion1 : DataTypeConversion
  Memory : Memory
  Relational Operator : RelationalOperator  Operator=~=  OutDataTypeStr=boolean
  Sum of Elements : Sum  Inputs=+
  OUT : Outport
  wires:
  Sum of Elements/1 -> Data Type Conversion1/1
  IN/1 -> Memory/1, Relational Operator/2
  Memory/1 -> Relational Operator/1
  Relational Operator/1 -> Data Type Conversion/1
  Data Type Conversion/1 -> Sum of Elements/1
  Data Type Conversion1/1 -> OUT/1

== system stepRecovery_compatibility/DesValues/State Machine Step Recovery/Step Recovery reference generator/Inverse Kinematics/Pseudo-Inverse kinematics Solver/ikin_DoubleIntegrator/Changed1 ==
  note: If the vector changes this block outputs 1, 0 otherwise
  IN : Inport
  Data Type Conversion : DataTypeConversion
  Data Type Conversion1 : DataTypeConversion
  Memory : Memory
  Relational Operator : RelationalOperator  Operator=~=  OutDataTypeStr=boolean
  Sum of Elements : Sum  Inputs=+
  OUT : Outport
  wires:
  Sum of Elements/1 -> Data Type Conversion1/1
  IN/1 -> Memory/1, Relational Operator/2
  Memory/1 -> Relational Operator/1
  Relational Operator/1 -> Data Type Conversion/1
  Data Type Conversion/1 -> Sum of Elements/1
  Data Type Conversion1/1 -> OUT/1

== system stepRecovery_compatibility/DesValues/State Machine Step Recovery/Step Recovery reference generator/Inverse Kinematics/Pseudo-Inverse kinematics Solver/ikin_utilities/ikin_Jacobians ==
  qRef_iKin : Inport
  Demux : Demux  Outputs=[16;ROBOT_DOF]
  Jacobian CoM : WBToolboxLibrary/wholeBodyModel/Jacobians/Jacobian  frameName='com'  robotName=WBT_robotName  localName=WBT_modelName  wbiFile=WBT_wbiFilename  wbiList=WBT_wbiList
  Jacobian l_foot : WBToolboxLibrary/wholeBodyModel/Jacobians/Jacobian  frameName='l_sole'  robotName=WBT_robotName  localName=WBT_modelName  wbiFile=WBT_wbiFilename  wbiList=WBT_wbiList
  Jacobian r_foot : WBToolboxLibrary/wholeBodyModel/Jacobians/Jacobian  frameName='r_sole'  robotName=WBT_robotName  localName=WBT_modelName  wbiFile=WBT_wbiFilename  wbiList=WBT_wbiList
  Reshape : Reshape  OutputDimensionality=Customize  OutputDimensions=[4,4]
  Jlsole : Outport
  Jrsole : Outport  Port=2
  JCoM : Outport  Port=3
  wires:
  qRef_iKin/1 -> Demux/1
  Demux/1 -> Reshape/1
  Reshape/1 -> Jacobian CoM/1, Jacobian r_foot/1, Jacobian l_foot/1
  Demux/2 -> Jacobian CoM/2, Jacobian r_foot/2, Jacobian l_foot/2
  Jacobian l_foot/1 -> Jlsole/1
  Jacobian r_foot/1 -> Jrsole/1
  Jacobian CoM/1 -> JCoM/1

== system stepRecovery_compatibility/DesValues/State Machine Step Recovery/Step Recovery reference generator/Inverse Kinematics/Pseudo-Inverse kinematics Solver/ikin_utilities/ikin_dJNu ==
  NuRef_iKin : Inport
  qRef_iKin : Inport  Port=2
  Demux : Demux  Outputs=[16;ROBOT_DOF]
  Demux1 : Demux  Outputs=[6;ROBOT_DOF]
  DotJ Nu CoM : WBToolboxLibrary/wholeBodyModel/Jacobians/DotJ Nu  frameName='com'  robotName=WBT_robotName  localName=WBT_modelName  wbiFile=WBT_wbiFilename  wbiList=WBT_wbiList
  DotJ Nu Left foot : WBToolboxLibrary/wholeBodyModel/Jacobians/DotJ Nu  frameName='l_sole'  robotName=WBT_robotName  localName=WBT_modelName  wbiFile=WBT_wbiFilename  wbiList=WBT_wbiList
  DotJ Nu Right foot : WBToolboxLibrary/wholeBodyModel/Jacobians/DotJ Nu  frameName='r_sole'  robotName=WBT_robotName  localName=WBT_modelName  wbiFile=WBT_wbiFilename  wbiList=WBT_wbiList
  Reshape5 : Reshape  OutputDimensionality=Customize  OutputDimensions=[4,4]
  dJlfootNu : Outport
  dJrfootNu : Outport  Port=2
  dJCoMNu : Outport  Port=3
  wires:
  Demux1/1 -> DotJ Nu Right foot/3, DotJ Nu Left foot/3, DotJ Nu CoM/3
  Demux/1 -> Reshape5/1
  Reshape5/1 -> DotJ Nu CoM/1, DotJ Nu Right foot/1, DotJ Nu Left foot/1
  DotJ Nu CoM/1 -> dJCoMNu/1
  DotJ Nu Right foot/1 -> dJrfootNu/1
  DotJ Nu Left foot/1 -> dJlfootNu/1
  NuRef_iKin/1 -> Demux1/1
  qRef_iKin/1 -> Demux/1
  Demux/2 -> DotJ Nu Right foot/2, DotJ Nu Left foot/2, DotJ Nu CoM/2
  Demux1/2 -> DotJ Nu Right foot/4, DotJ Nu Left foot/4, DotJ Nu CoM/4

== system stepRecovery_compatibility/DesValues/State Machine Step Recovery/Step Recovery reference generator/Inverse Kinematics/Pseudo-Inverse kinematics Solver/ikin_utilities/ikin_forwardKin ==
  qRef_iKin_init : Inport
  qRef_iKin : Inport  Port=2
  lsole_H_rsole : Inport  Port=3
  "rsole_H_lsole " : Inport  Port=4
  Demux1 : Demux  Outputs=[16;ROBOT_DOF]
  Demux2 : Demux  Outputs=[16;ROBOT_DOF]
  Forward KinematicsCoM : WBToolboxLibrary/wholeBodyModel/Kinematics/Forward Kinematics  frameName='com'  robotName=WBT_robotName  localName=WBT_modelName  wbiFile=WBT_wbiFilename  wbiList=WBT_wbiList
  Forward Kinematics_lFoot : WBToolboxLibrary/wholeBodyModel/Kinematics/Forward Kinematics  frameName='l_sole'  robotName=WBT_robotName  localName=WBT_modelName  wbiFile=WBT_wbiFilename  wbiList=WBT_wbiList
  Forward Kinematics_lFoot_init : WBToolboxLibrary/wholeBodyModel/Kinematics/Forward Kinematics  frameName='l_sole'  robotName=WBT_robotName  localName=WBT_modelName  wbiFile=WBT_wbiFilename  wbiList=WBT_wbiList
  Forward Kinematics_rFoot : WBToolboxLibrary/wholeBodyModel/Kinematics/Forward Kinematics  frameName='r_sole'  robotName=WBT_robotName  localName=WBT_modelName  wbiFile=WBT_wbiFilename  wbiList=WBT_wbiList
  Forward Kinematics_rFoot_init : WBToolboxLibrary/wholeBodyModel/Kinematics/Forward Kinematics  frameName='r_sole'  robotName=WBT_robotName  localName=WBT_modelName  wbiFile=WBT_wbiFilename  wbiList=WBT_wbiList
  FromFwdKin_ToPosAndOrient : MATLAB Function  TreatAsAtomicUnit=on
      settings: PermitHierarchicalResolution=ParametersOnly
  Reshape1 : Reshape  OutputDimensionality=Customize  OutputDimensions=[4,4]
  Reshape2 : Reshape  OutputDimensionality=Customize  OutputDimensions=[4,4]
  CoMpos : Outport
  deltaLFootPos : Outport  Port=2
  deltaRFootOri : Outport  Port=3
  deltaRFootPos : Outport  Port=4
  deltaLFootOri : Outport  Port=5
  cartesian_err : Outport  Port=6
  wires:
  qRef_iKin_init/1 -> Demux2/1
  Demux2/1 -> Reshape1/1
  qRef_iKin/1 -> Demux1/1
  Demux1/1 -> Reshape2/1
  Reshape2/1 -> Forward KinematicsCoM/1, Forward Kinematics_rFoot/1, Forward Kinematics_lFoot/1
  Reshape1/1 -> Forward Kinematics_lFoot_init/1, Forward Kinematics_rFoot_init/1
  Demux2/2 -> Forward Kinematics_lFoot_init/2, Forward Kinematics_rFoot_init/2
  Demux1/2 -> Forward KinematicsCoM/2, Forward Kinematics_lFoot/2, Forward Kinematics_rFoot/2
  Forward Kinematics_lFoot/1 -> FromFwdKin_ToPosAndOrient/1(fwdkin_lfoot)
  Forward Kinematics_rFoot/1 -> FromFwdKin_ToPosAndOrient/2(fwdkin_rfoot)
  Forward KinematicsCoM/1 -> FromFwdKin_ToPosAndOrient/3(fwdkinCoM)
  Forward Kinematics_rFoot_init/1 -> FromFwdKin_ToPosAndOrient/4(fwdkin_rfootIni)
  Forward Kinematics_lFoot_init/1 -> FromFwdKin_ToPosAndOrient/5(fwdkin_lfootIni)
  FromFwdKin_ToPosAndOrient/5(CoMPos) -> CoMpos/1
  FromFwdKin_ToPosAndOrient/1(delta_lfootPos) -> deltaLFootPos/1
  FromFwdKin_ToPosAndOrient/2(delta_lfootOri) -> deltaLFootOri/1
  FromFwdKin_ToPosAndOrient/3(delta_rfootPos) -> deltaRFootPos/1
  FromFwdKin_ToPosAndOrient/4(delta_rfootOri) -> deltaRFootOri/1
  lsole_H_rsole/1 -> FromFwdKin_ToPosAndOrient/6(lsole_H_rsole)
  "rsole_H_lsole "/1 -> FromFwdKin_ToPosAndOrient/7(rsole_H_lsole)
  FromFwdKin_ToPosAndOrient/6(cartesian_err) -> cartesian_err/1

== system stepRecovery_compatibility/DesValues/State Machine Step Recovery/Step Recovery reference generator/Inverse Kinematics/Pseudo-Inverse kinematics Solver/q+base/Changed1 ==
  note: If the vector changes this block outputs 1, 0 otherwise
  IN : Inport
  Data Type Conversion : DataTypeConversion
  Data Type Conversion1 : DataTypeConversion
  Memory : Memory
  Relational Operator : RelationalOperator  Operator=~=  OutDataTypeStr=boolean
  Sum of Elements : Sum  Inputs=+
  OUT : Outport
  wires:
  Sum of Elements/1 -> Data Type Conversion1/1
  IN/1 -> Memory/1, Relational Operator/2
  Memory/1 -> Relational Operator/1
  Relational Operator/1 -> Data Type Conversion/1
  Data Type Conversion/1 -> Sum of Elements/1
  Data Type Conversion1/1 -> OUT/1

== system stepRecovery_compatibility/DesValues/State Machine Step Recovery/Step Recovery reference generator/Step Recovery Techniques /Capture Point Computer/Capture Point/omega ==
  COMx : Inport
  Constant : Constant  Value=9.81
  Divide : Product  Inputs=*/
  Selector : Selector  InputPortWidth=3  IndexOptions=Index vector (dialog)  Indices=[3]  OutputSizes=1
  Sqrt : Sqrt  SaturateOnIntegerOverflow=on
  holder 1 : WBToolboxLibrary/Utilities/holder 
  omega : Outport
  wires:
  COMx/1 -> Selector/1
  Selector/1 -> holder 1/1
  holder 1/1 -> Divide/2
  Constant/1 -> Divide/1
  Divide/1 -> Sqrt/1
  Sqrt/1 -> omega/1

== system stepRecovery_compatibility/DesValues/State Machine Step Recovery/Step Recovery reference generator/Step Recovery Techniques /Capture Point Computer/Capture Point-Pratt /omega ==
  COMx : Inport
  Constant : Constant  Value=9.81
  Divide : Product  Inputs=*/
  Selector : Selector  InputPortWidth=3  IndexOptions=Index vector (dialog)  Indices=[3]  OutputSizes=1
  Sqrt : Sqrt  SaturateOnIntegerOverflow=on
  holder 1 : WBToolboxLibrary/Utilities/holder 
  omega : Outport
  wires:
  COMx/1 -> Selector/1
  Selector/1 -> holder 1/1
  holder 1/1 -> Divide/2
  Constant/1 -> Divide/1
  Divide/1 -> Sqrt/1
  Sqrt/1 -> omega/1
